simulink model "impedance_measurement"  (R2019a)
settings: Solver=VariableStepAuto  StartTime=0.0  StopTime=1e-4  RelTol=1e-3
libraries: fl_lib x6, nesl_utility x3, powerlib_meascontrol x2, ee_lib x1
settings Model: Creator=vadim.piskun  LastModifiedBy=prakhark

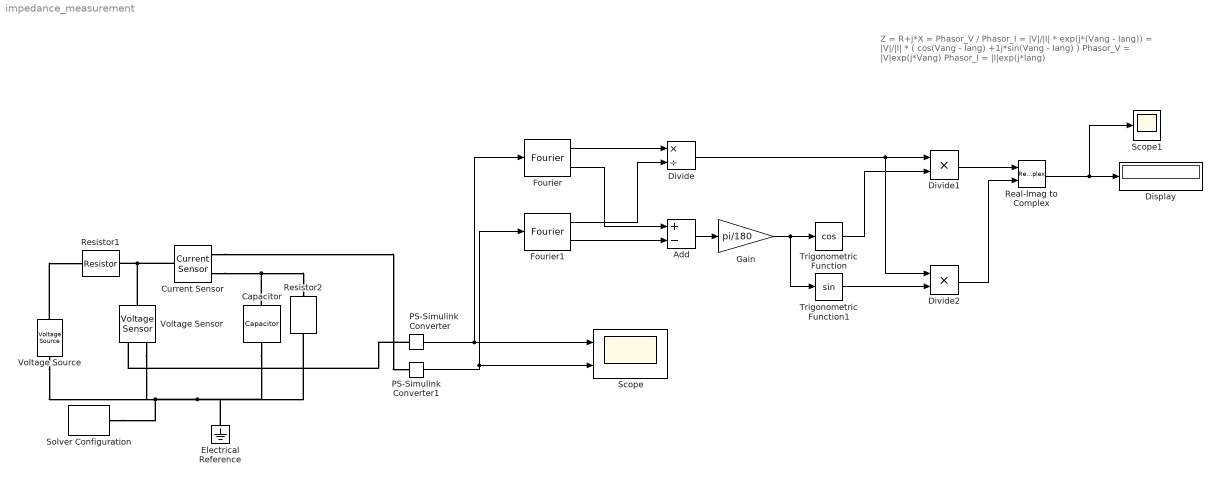
== system impedance_measurement ==
  note: Z = R+j*X = Phasor_V / Phasor_I = |V|/|I| * exp(j*(Vang - Iang))
      | =  |V|/|I| * ( cos(Vang - Iang) +1j*sin(Vang - Iang)     )
      |
      | Phasor_V = |V|exp(j*Vang)
      | Phasor_I = |I|exp(j*Iang)
  Add : Sum  Inputs=+-
  Capacitor : fl_lib/Electrical/Electrical Elements/Capacitor  c=1e-6 F  r=1e-6 Ohm  g=0 1/Ohm  i_specify=off  i_priority=None  i=0 A  i_nominal_specify=off  i_nominal_unit=A  i_nominal_value=1  v_specify=off  v_priority=None  v=0 V  v_nominal_specify=off  v_nominal_unit=V  v_nominal_value=1  vc_specify=off  vc_priority=High  vc=0 V  vc_nominal_specify=off  vc_nominal_unit=V  vc_nominal_value=1
  Current Sensor : fl_lib/Electrical/Electrical Sensors/Current Sensor
  Display : Display
  Divide : Product  Inputs=*/
  Divide1 : Product  Inputs=**
  Divide2 : Product  Inputs=**
  Electrical Reference : fl_lib/Electrical/Electrical Elements/Electrical Reference
  Fourier : powerlib_meascontrol/Measurements/Fourier  Freq=100e3  n=1  InInit=[0, 0]  Ts=1e-8
      settings: SourceProductName=Simscape Electrical
  Fourier1 : powerlib_meascontrol/Measurements/Fourier  Freq=100e3  n=1  InInit=[0.1, 0]  Ts=1e-8
      settings: SourceProductName=Simscape Electrical
  Gain : Gain  Gain=pi/180
  PS-Simulink Converter : nesl_utility/PS-Simulink Converter  PhysicalDomain=network_engine_domain  SubClassName=ps_output  LeftPortType=input  RightPortType=output  PseudoPeriodic=off  Frequencies=[]  Unit=1  AffineConversion=off
  PS-Simulink Converter1 : nesl_utility/PS-Simulink Converter  PhysicalDomain=network_engine_domain  SubClassName=ps_output  LeftPortType=input  RightPortType=output  PseudoPeriodic=off  Frequencies=[]  Unit=1  AffineConversion=off
  Real-Imag to Complex : RealImagToComplex
  Resistor1 : fl_lib/Electrical/Electrical Elements/Resistor  R=50 Ohm  i_specify=off  i_priority=None  i=0 A  i_nominal_specify=off  i_nominal_unit=A  i_nominal_value=1  v_specify=off  v_priority=None  v=0 V  v_nominal_specify=off  v_nominal_unit=V  v_nominal_value=1
  Resistor2 : fl_lib/Electrical/Electrical Elements/Resistor  R=50 Ohm  i_specify=off  i_priority=None  i=0 A  i_nominal_specify=off  i_nominal_unit=A  i_nominal_value=1  v_specify=off  v_priority=None  v=0 V  v_nominal_specify=off  v_nominal_unit=V  v_nominal_value=1
  Scope : Scope  NumInputPorts=2
  Scope1 : Scope
  Solver Configuration : nesl_utility/Solver Configuration  PhysicalDomain=network_engine_domain  SubClassName=solver  LeftPortType=input  RightPortType=generic  Tones=[]  Harmonics=[]  SimulateNoise=off  Profile=off  UseLocalSampling=off  EnableSwitchedLinearOptims=on  FrequencyDomain=off  UseCCode=off  RelTol=0.001  AbsTol=1e-06  MinStep=1e-09  ToWorkspace=off  RevertToSquareIcSolve=off  NumHomotopyIterations=100  PhasorMode=off  PhasorModeNumHarmonics=1  DoDC=off  ResidualTolerance=1e-09  UseLocalSolver=on  LocalSolverChoice=NE_BACKWARD_EULER_ADVANCER  LocalSolverSampleTime=1e-8  DoFixedCost=on  MaxNonlinIter=3  MaxModeIter=2  LinearAlgebra=auto  EquationFormulation=NE_TIME_EF  DelaysMemoryBudget=1024  AutomaticFiltering=on  FilteringTimeConstant=0.001  PartitionStorageMethod=AS_NEEDED  PartitionMemoryBudget=1024  PartitionMethod=ROBUST
  Trigonometric Function : Trigonometry  Operator=cos
  Trigonometric Function1 : Trigonometry
  Voltage Sensor : fl_lib/Electrical/Electrical Sensors/Voltage Sensor
  Voltage Source : ee_lib/Sources/Voltage Source  dc_voltage=0 V  ac_voltage=10 V  ac_shift=0 rad  ac_frequency=100 kHz  noise_mode=0  PSD=0 V^2/Hz  repeatability=1  auto_seed=2003653836  user_seed=0  sample_time=1e-3 s  i_specify=off  i_priority=None  i=0 A  i_nominal_specify=off  i_nominal_unit=A  i_nominal_value=1  v_specify=off  v_priority=None  v=0 V  v_nominal_specify=off  v_nominal_unit=V  v_nominal_value=1
      settings: SourceProductName=Simscape Electrical
  wires:
  PS-Simulink Converter/1 -> Fourier/1, Scope/1
  PS-Simulink Converter1/1 -> Fourier1/1, Scope/2
  Fourier/1 -> Divide/1
  Fourier1/1 -> Divide/2
  Fourier/2 -> Add/1
  Fourier1/2 -> Add/2
  Add/1 -> Gain/1
  Gain/1 -> Trigonometric Function1/1, Trigonometric Function/1
  Divide/1 -> Divide2/1, Divide1/1
  Trigonometric Function/1 -> Divide1/2
  Trigonometric Function1/1 -> Divide2/2
  Divide1/1 -> Real-Imag to Complex/1
  Divide2/1 -> Real-Imag to Complex/2
  Real-Imag to Complex/1 -> Scope1/1, Display/1
  connections:
  Solver Configuration/RConn1 -- Electrical Reference/LConn1 -- Capacitor/RConn1 -- Resistor2/RConn1 -- Voltage Sensor/RConn2 -- Voltage Source/RConn1
  Voltage Source/LConn1 -- Resistor1/RConn1
  Voltage Sensor/LConn1 -- Current Sensor/LConn1 -- Resistor1/LConn1
  PS-Simulink Converter/LConn1 -- Voltage Sensor/RConn1
  Current Sensor/RConn2 -- Capacitor/LConn1 -- Resistor2/LConn1
  Current Sensor/RConn1 -- PS-Simulink Converter1/LConn1
